simulink model "SoftwareSystemArchitecture"  (R2016b)
settings: Solver=FixedStepAuto  StartTime=0.0  StopTime=10.0  RelTol=1e-3
settings Model: Creator=NEATdemo  LastModifiedBy=NEATdemo

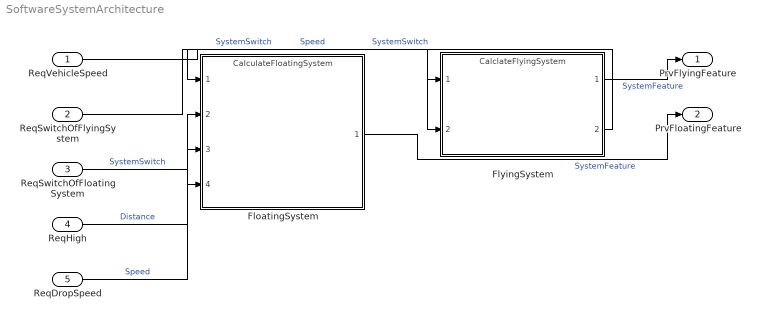
== system SoftwareSystemArchitecture ==
  ReqVehicleSpeed : Inport
      settings: AttributesFormatString=Speed
  ReqSwitchOfFlyingSystem : Inport  Port=2
      settings: AttributesFormatString=SystemSwitch
  ReqSwitchOfFloatingSystem : Inport  Port=3
      settings: AttributesFormatString=SystemSwitch
  ReqHigh : Inport  Port=4
      settings: AttributesFormatString=Distance
  ReqDropSpeed : Inport  Port=5
      settings: AttributesFormatString=Speed
  FloatingSystem : ModelReference  ModelNameDialog=CalculateFloatingSystem  SimulationMode=Normal  ModelReferenceVersion=1.9
  FlyingSystem : ModelReference  ModelNameDialog=CalclateFlyingSystem  SimulationMode=Normal  ModelReferenceVersion=1.8
  PrvFlyingFeature : Outport
      settings: AttributesFormatString=SystemFeature
  PrvFloatingFeature : Outport  Port=2
      settings: AttributesFormatString=SystemFeature
  wires:
  FlyingSystem/2 -> FloatingSystem/1  "SystemSwitch"
  ReqVehicleSpeed/1 -> FlyingSystem/2  "Speed"
  ReqSwitchOfFlyingSystem/1 -> FlyingSystem/1  "SystemSwitch"
  FlyingSystem/1 -> PrvFlyingFeature/1  "SystemFeature"
  ReqSwitchOfFloatingSystem/1 -> FloatingSystem/2  "SystemSwitch"
  ReqHigh/1 -> FloatingSystem/3  "Distance"
  ReqDropSpeed/1 -> FloatingSystem/4  "Speed"
  FloatingSystem/1 -> PrvFloatingFeature/1  "SystemFeature"
